simulink model "r08_esame2013mod_b"  (Simulink 7.9)
settings: Solver=ode45  StartTime=0.0  StopTime=5  MaxStep=0.1  RelTol=1e-3  AbsTol=1e-3
values from neighbouring files (symbols this model uses):
  A = [1 2;1 0]    [esame2013_a.m]    (also in esame2013_b.m = [41 81;-20 -40], eigA = eig(A))
  B = [1; 0]    [esame2013_a.m]    (also in esame2013_b.m = [1; 1])
  C = [.5 1]    [esame2013_a.m]    (also in esame2013_b.m = [6 11])
  K = place(A,B,autoval)    [esame2013_a.m]    (also in esame2013_b.m)
  L = place(A', C', avals_puntoc)'    [esame2013_b.m]
  x0 = [0; 0]    [esame2013_a.m]    (also in esame2013_b.m)
  xEQ = [0; 0]    [esame2013_a.m]    (also in esame2013_b.m)
undefined symbols (not defined in the file or in its folder): sigbuilder_block
settings Model: Creator=claudio  LastModifiedBy=patrizio  ExtModeTrigMode=oneshot  ExtModeArmWhenConnect=off
settings DataIOCC: LimitDataPoints=off  SaveOutput=off  SaveTime=off
settings OptimizationCC: BooleanDataType=off  InlineInvariantSignals=on  InitFltsAndDblsToZero=on
settings DebuggingCC: SaveWithParameterizedLinksMsg=none  SignalResolutionControl=TryResolveAllWithWarning  SolverPrmCheckMsg=none  MultiTaskDSMMsg=warning  MultiTaskCondExecSysMsg=none  FcnCallInpInsideContextMsg=Use local settings  StrictBusMsg=None
settings HardwareCC: TargetUnknown=on
settings RTWCC: IncludeERTFirstTime=on
settings GRTTargetCC: TargetFcnLib=ansi_tfl_tmw.mat  ModelReferenceCompliant=off  CombineOutputUpdateFcns=off  MatFileLogging=off  GRTInterface=on

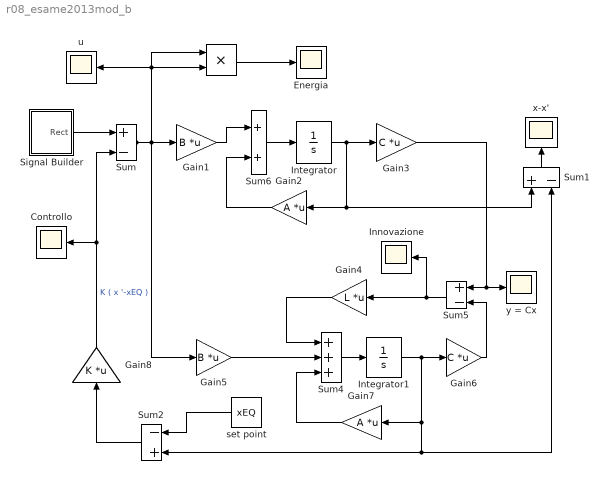
== system r08_esame2013mod_b ==
  "     " : Product  RndMeth=Zero
  Controllo : Scope
      settings: TimeRange=5  YMin=-100  YMax=200  SaveName=ScopeData3
  Energia : Scope
      settings: TimeRange=20  SaveName=ScopeData7
  Gain1 : Gain  Gain=B  Multiplication=Matrix(K*u)
  Gain2 : Gain  Gain=A  Multiplication=Matrix(K*u)
  Gain3 : Gain  Gain=C  Multiplication=Matrix(K*u)
  Gain4 : Gain  Gain=L  Multiplication=Matrix(K*u)
  Gain5 : Gain  Gain=B  Multiplication=Matrix(K*u)
  Gain6 : Gain  Gain=C  Multiplication=Matrix(K*u)
  Gain7 : Gain  Gain=A  Multiplication=Matrix(K*u)
  Gain8 : Gain  Gain=K  Multiplication=Matrix(K*u)
  Innovazione : Scope
      settings: SaveName=ScopeData4
  Integrator : Integrator  InitialCondition=x0
  Integrator1 : Integrator  InitialCondition=[ 0 0 ]
  Signal Builder : Subsystem  Tag=STV Subsys  LoadFcn=sigbuilder_block('load');  StartFcn=sigbuilder_block('start');  StopFcn=sigbuilder_block('stop');  ClipboardFcn=sigbuilder_block('clipboard');  mask(Sigbuilder block){}
      mask help: Sigbuilder GUI
      mask init:
      | if ~strcmp(get_param(bdroot(gcbh),'SimulationStatus'),'stopped') tuvar = sigbuilder_block('maskInit'); end
      settings: CopyFcn=sigbuilder_block('copy');  DeleteFcn=sigbuilder_block('delete');  ModelCloseFcn=sigbuilder_block('modelClose');  PreSaveFcn=sigbuilder_block('preSave');  PauseFcn=sigbuilder_block('pause')  ContinueFcn=sigbuilder_block('continue')  NameChangeFcn=sigbuilder_block('namechange');  OpenFcn=sigbuilder_block('open',[289.6 112.8 520 400 ]);  CloseFcn=sigbuilder_block('close');
      mask Display: plot(0,0,100,100,[10,10,40,40,10],[80,20,20,80,80],[40,10],[50,50], [40,27,10],[65,72,56],[40,25,25,10],[28,28,43,43]);
  Sum : Sum  Inputs=+-  SaturateOnIntegerOverflow=on  InputSameDT=on  OutDataTypeStr=Inherit: Same as first input
  Sum1 : Sum  Inputs=+-  SaturateOnIntegerOverflow=on  InputSameDT=on  OutDataTypeStr=Inherit: Same as first input
  Sum2 : Sum  Inputs=-+  SaturateOnIntegerOverflow=on  InputSameDT=on  OutDataTypeStr=Inherit: Same as first input
  Sum4 : Sum  Inputs=+++  SaturateOnIntegerOverflow=on  InputSameDT=on  OutDataTypeStr=Inherit: Same as first input
  Sum5 : Sum  Inputs=+-  SaturateOnIntegerOverflow=on  InputSameDT=on  OutDataTypeStr=Inherit: Same as first input
  Sum6 : Sum  SaturateOnIntegerOverflow=on  InputSameDT=on  OutDataTypeStr=Inherit: Same as first input
  set point : Constant  Value=xEQ
  u : Scope
      settings: TimeRange=20  SaveName=ScopeData8
  x-x' : Scope
      settings: TimeRange=10
  y = Cx : Scope
      settings: TimeRange=20  YMin=-1  YMax=1  SaveName=ScopeData6
  wires:
  Integrator1/1 -> Gain7/1, Sum1/2, Sum2/2, Gain6/1
  Sum4/1 -> Integrator1/1
  Gain7/1 -> Sum4/3
  Gain5/1 -> Sum4/2
  Gain3/1 -> Sum5/1, y = Cx/1
  Gain6/1 -> Sum5/2
  Gain4/1 -> Sum4/1
  Integrator/1 -> Gain3/1, Gain2/1, Sum1/1
  Sum5/1 -> Gain4/1, Innovazione/1
  Sum6/1 -> Integrator/1
  Gain8/1 -> Sum/2, Controllo/1  "K ( x '-xEQ )"
  Gain2/1 -> Sum6/2
  Sum/1 -> Gain1/1, Gain5/1, "     "/1, "     "/2, u/1
  Sum1/1 -> x-x'/1
  set point/1 -> Sum2/1
  Sum2/1 -> Gain8/1
  Signal Builder/1(Rect) -> Sum/1
  "     "/1 -> Energia/1
  Gain1/1 -> Sum6/1

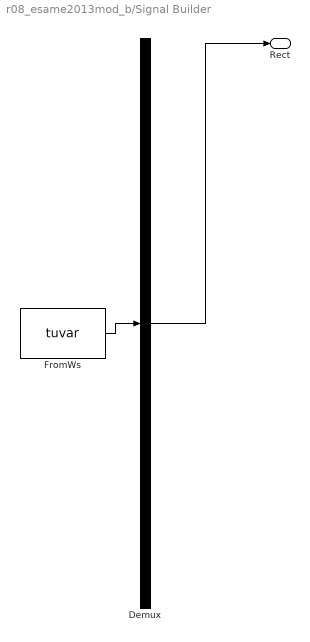
== system r08_esame2013mod_b/Signal Builder ==
  Demux : Demux  Tag=STV Demux  Outputs=1
  FromWs : FromWorkspace  Tag=STV FromWs  VariableName=tuvar  SampleTime=0  SigBuilderData=DataTag0  VnvData=DataTag1
      SigBuilderData=|
      | dataSet.timeRange = [0 10]
      | dataSet.name = 'Group 1'
      | sbobj.Name = 'Signal Builder'
      | sbobj.Groups.Name = 'Group 1'
      | sbobj.Groups.Signals.Name = 'Rect'
      | sbobj.Groups.Signals.XData = [0 1 2 2 3 3 10]
      | sbobj.Groups.Signals.YData = [0 0 0 4 4 0 0]
  Rect : Outport  Tag=STV Outport
  wires:
  Demux/1 -> Rect/1
  FromWs/1 -> Demux/1
